simulink model "dng_aircraft_demo"  (Simulink 5.0)
settings: Solver=ode45  StartTime=0.0  StopTime=inf  MaxStep=0.1  RelTol=1e-2  AbsTol=1e-3
PreLoadFcn:
  | load dng_aircraft_init;
values from neighbouring files (symbols this model uses):
  AM = [-0.03554 -0.002226 -0.05504 0.000591 0.09448 -0.003117 0.00292 0 -5.578 0 -0.6028 0 ... (114 elements, 6x19)]    [dng_aircraft_init.mat]
  GM1 = [1.5875 14.63 23.23 5368.39 6928.93 11158.75 0 117.64 0 2288.231]    [dng_aircraft_init.mat]
  uaero0 = [-0.0317656979071 -0.0320210159663 -0.0365180369264 0]    [dng_aircraft_init.mat]
  uprop0 = [1800 22.5734756773]    [dng_aircraft_init.mat]
  xfix = 1    [dng_aircraft_init.mat]
  xinco = [45 0.13029612885 0.0603452248515 0 0 0 0 0.13029612885 0 0 0 1000]    [dng_aircraft_init.mat]
undefined symbols (not defined in the file or in its folder): tcinclinometer, tcturn, xpos, ypos, zpos
libraries: dnglibv1 x10
settings Model: Creator=nikita  LastModifiedBy=howie  ExtModeTrigMode=oneshot  ExtModeArmWhenConnect=off  LimitDataPoints=off  IntegerOverflowMsg=none  BlockReductionOpt=off  BooleanDataType=off
settings Model: ModifiedHistory=|
  | March 03, 1999:
  | Fine-tuned control parameters. Included rate-limiter in flap-signal.
  | Included 1st-order lag filter in vertical speed signal. - Marc Rauw.

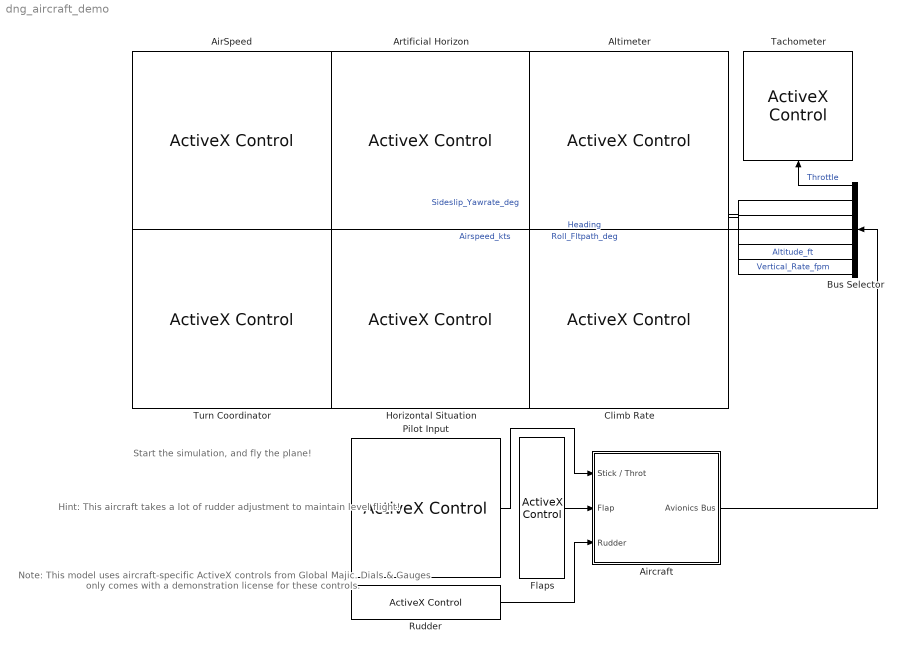
== system dng_aircraft_demo ==
  note: Note: This model uses
      | aircraft-specific ActiveX
      | controls from Global Majic.
      | Dials & Gauges only comes
      | with a demonstration
      | license for these controls.
  note: Start the simulation,
      | and fly the plane!
  note: Hint: This aircraft takes a
      | lot of rudder adjustment
      | to maintain level flight!
  AirSpeed : dnglibv1/ActiveX Control  Orientation=up  progid=air.airctrl.1  connect=input  input=airspeed  init=hActx.displaymode=4;  inblock=on  border=off  dialOut=0  updateParam=0
  Aircraft : Subsystem
  Altimeter : dnglibv1/ActiveX Control  Orientation=up  progid=air.airctrl.1  connect=input  input=altitude  init=hActx.displaymode=2;hActx.altthousandstyle=1;  inblock=on  border=off  dialOut=0  updateParam=0
  Artificial Horizon : dnglibv1/ActiveX Control  Orientation=up  progid=air.airctrl.1  connect=input  input=ahroll, ahpitch  init=hActx.displaymode=6;  inblock=on  border=off  dialOut=0  updateParam=0
  Bus Selector : BusSelector  Orientation=left  OutputSignals=Throttle,Avionics.Airspeed_kts,Avionics.Roll_Fltpath_deg,Avionics.Sideslip_Yawrate_deg,Avionics.Heading,Avionics.Altitude_ft,Avionics.Vertical_Rate_fpm
  Climb Rate : dnglibv1/ActiveX Control  Orientation=down  progid=air.airctrl.1  connect=input  input=climbrate  init=hActx.displaymode=3;  inblock=on  border=off  dialOut=0  updateParam=0
  Flaps : dnglibv1/ActiveX Control  progid=mwslider.sliderctrl.1  connect=output  output=value  dialOutEvent=Slide  init=hActx.configuration='Slider\Basic\Vertical\Simple Slider 3';dng_aircraft_set_flap(hActx);  inblock=on  border=off  dialOut=1  updateParam=0
  Horizontal Situation : dnglibv1/ActiveX Control  Orientation=down  progid=air.airctrl.1  connect=input  input=hsiheading  init=hActx.displaymode=5;  inblock=on  border=off  dialOut=0  updateParam=0
  Pilot Input : dnglibv1/ActiveX Control  progid=JOYSTICK.JoystickCtrl.1  connect=output  output=ypos,xpos,zpos  dialOutEvent=JoyMove  init=hActx.displaymode=1;hActx.ymax=-9; hActx.ymin=9; hActx.xmax=-18;hActx.xmin=18;hActx.zmin=2600; hActx.zmax=1100;hActx.zpos=1800;  inblock=on  border=off  dialOut=[0.000176597852259874;1.4586243135349e-019;1800]  updateParam=0
  Rudder : dnglibv1/ActiveX Control  progid=mwslider.sliderctrl.1  connect=output  output=value  dialOutEvent=Slide  init=hActx.configuration='Slider\Basic\Horizontal\Simple Slider3';hActx.min=-5;hActx.max=5;hActx.value=0;  inblock=on  border=off  dialOut=0  updateParam=0
  Tachometer : dnglibv1/ActiveX Control  Orientation=up  progid=mwagauge.agaugectrl.1  connect=input  input=NeedleValue  init=hActx.configuration='Angular Gauge\Automobile Instruments\Engine RPM';hActx.scalemaxvalue=5000;hActx.Tics=1;hActx.TicAutoTic=1;hActx.TicAutoCount=4;hActx.Captions=1;hActx.Caption='RPM';  inblock=on  border=off  dialOut=0  updateParam=0
  Turn Coordinator : dnglibv1/ActiveX Control  Orientation=down  progid=air.airctrl.1  connect=input  input=tcinclinometer,tcturn  init=hActx.displaymode=7;  inblock=on  border=off  dialOut=0  updateParam=0
  wires:
  Aircraft/1(Avionics Bus) -> Bus Selector/1
  Bus Selector/2 -> AirSpeed/1  "Airspeed_kts"
  Bus Selector/3 -> Artificial Horizon/1  "Roll_Fltpath_deg"
  Bus Selector/5 -> Horizontal Situation/1  "Heading"
  Bus Selector/6 -> Altimeter/1  "Altitude_ft"
  Bus Selector/7 -> Climb Rate/1  "Vertical_Rate_fpm"
  Pilot Input/1 -> Aircraft/1(Stick / Throt)
  Rudder/1 -> Aircraft/3(Rudder)
  Flaps/1 -> Aircraft/2(Flap)
  Bus Selector/4 -> Turn Coordinator/1  "Sideslip_Yawrate_deg"
  Bus Selector/1 -> Tachometer/1  "Throttle"

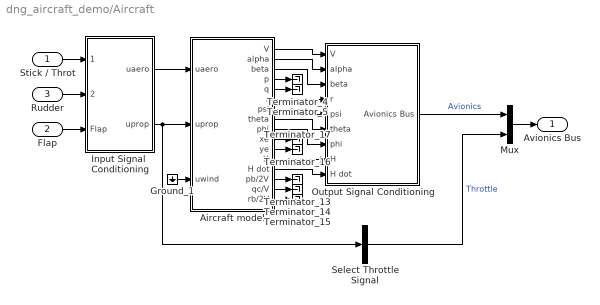
== system dng_aircraft_demo/Aircraft ==
  Stick / Throt : Inport
  Flap : Inport  Port=2
  Rudder : Inport  Port=3
  Aircraft model : Subsystem
  Ground_1 : Ground
  Input Signal  Conditioning : Subsystem
  Mux : Mux  Inputs=2
  Output Signal Conditioning : Subsystem
  Select Throttle Signal : BusSelector  OutputSignals=Throttle
  Terminator_{4..5,13..17} (7 alike) : Terminator
  Avionics Bus : Outport
  wires:
  Input Signal  Conditioning/1(uaero) -> Aircraft model/1(uaero)
  Ground_1/1 -> Aircraft model/3(uwind)
  Stick / Throt/1 -> Input Signal  Conditioning/1(Stick / Throt)
  Rudder/1 -> Input Signal  Conditioning/2(Rudder)
  Flap/1 -> Input Signal  Conditioning/3(Flap)
  Aircraft model/4(p) -> Terminator_4/1
  Aircraft model/5(q) -> Terminator_5/1
  Aircraft model/10(xe) -> Terminator_16/1
  Aircraft model/11(ye) -> Terminator_17/1
  Aircraft model/14(pb/2V) -> Terminator_13/1
  Aircraft model/15(qc/V) -> Terminator_14/1
  Aircraft model/16(rb/2V) -> Terminator_15/1
  Aircraft model/1(V) -> Output Signal Conditioning/1(V)
  Aircraft model/2(alpha) -> Output Signal Conditioning/2(alpha)
  Aircraft model/3(beta) -> Output Signal Conditioning/3(beta)
  Aircraft model/6(r) -> Output Signal Conditioning/4(r)
  Aircraft model/7(psi) -> Output Signal Conditioning/5(psi)
  Aircraft model/8(theta) -> Output Signal Conditioning/6(theta)
  Aircraft model/9(phi) -> Output Signal Conditioning/7(phi)
  Aircraft model/12(H) -> Output Signal Conditioning/8(H)
  Aircraft model/13(H dot) -> Output Signal Conditioning/9(H dot)
  Mux/1 -> Avionics Bus/1
  Output Signal Conditioning/1(Avionics Bus) -> Mux/1  "Avionics"
  Input Signal  Conditioning/2(uprop) -> Aircraft model/2(uprop), Select Throttle Signal/1
  Select Throttle Signal/1 -> Mux/2  "Throttle"

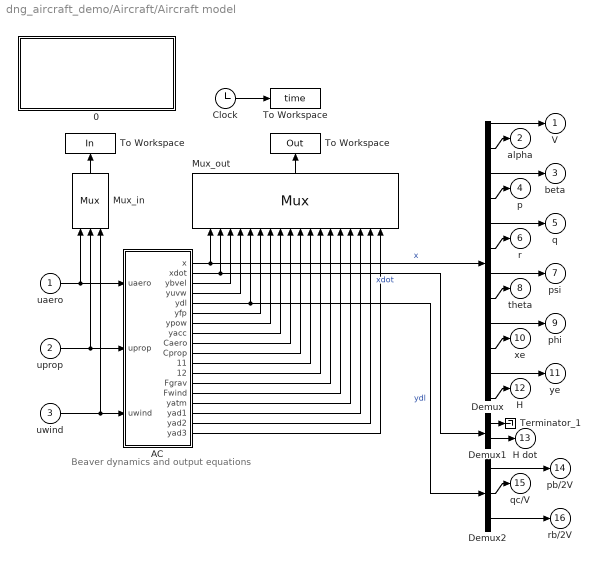
== system dng_aircraft_demo/Aircraft/Aircraft model ==
  note: Beaver dynamics
      | and output equations
  uaero : Inport  PortDimensions=4
  uprop : Inport  Port=2  PortDimensions=2
  uwind : Inport  Port=3  PortDimensions=6
  0 : Subsystem
      settings: OpenFcn=web('http://callisto.worldonline.nl/~rauw');
      mask Display: disp('Dynamic model of the\nDe Havilland DHC-2 ''Beaver'',\ncreated by M.O. Rauw.\nDouble-click for more info.')
  AC : Subsystem
  Clock : Clock
      settings: Decimation=10
  Demux : Demux  Outputs=12
  Demux1 : Demux  Outputs=[11 1]
  Demux2 : Demux  Outputs=3
  Mux_in : Mux  Orientation=up  Inputs=[4 2 6]
      settings: OpenFcn=web('http://callisto.worldonline.nl/~rauw');
      mask Display: disp('Mux\nClick\n2x for\ninfo!')
  Mux_out : Mux  Orientation=up  Inputs=[12 12 3 3 3 4 2 6 6 6 6 6 3 3 5 3 3 3]
      settings: OpenFcn=web('http://callisto.worldonline.nl/~rauw');
      mask Display: disp('Mux\n\nDouble-click for more info!')
  Terminator_1 : Terminator
  To Workspace : ToWorkspace  VariableName=Out  SaveFormat=Array
      settings: Orientation=up  MaxDataPoints=5000
  "To Workspace " : ToWorkspace  VariableName=In  SaveFormat=Array
      settings: Orientation=up  MaxDataPoints=5000
  "To Workspace  " : ToWorkspace  VariableName=time  SaveFormat=Array
      settings: MaxDataPoints=5000
  V : Outport  InitialOutput=0
  alpha : Outport  Port=2  InitialOutput=0
  beta : Outport  Port=3  InitialOutput=0
  p : Outport  Port=4  InitialOutput=0
  q : Outport  Port=5  InitialOutput=0
  r : Outport  Port=6  InitialOutput=0
  psi : Outport  Port=7  InitialOutput=0
  theta : Outport  Port=8  InitialOutput=0
  phi : Outport  Port=9  InitialOutput=0
  xe : Outport  Port=10  InitialOutput=0
  ye : Outport  Port=11  InitialOutput=0
  H : Outport  Port=12  InitialOutput=0
  H dot : Outport  Port=13  InitialOutput=0
  pb/2V : Outport  Port=14  InitialOutput=0
  qc/V : Outport  Port=15  InitialOutput=0
  rb/2V : Outport  Port=16  InitialOutput=0
  wires:
  uaero/1 -> Mux_in/1, AC/1(uaero)
  uprop/1 -> Mux_in/2, AC/2(uprop)
  uwind/1 -> Mux_in/3, AC/3(" uwind")
  AC/18(yad3) -> Mux_out/18
  AC/17(yad2) -> Mux_out/17
  AC/4(yuvw) -> Mux_out/4
  AC/1(x) -> Mux_out/1, Demux/1  "x"
  AC/3(ybvel) -> Mux_out/3
  AC/16(yad1) -> Mux_out/16
  AC/5(ydl) -> Mux_out/5, Demux2/1  "ydl"
  AC/6(yfp) -> Mux_out/6
  AC/8(yacc) -> Mux_out/8
  AC/9(Caero) -> Mux_out/9
  AC/10(Cprop) -> Mux_out/10
  AC/11(FMaero) -> Mux_out/11
  AC/12(FMprop) -> Mux_out/12
  AC/13(Fgrav) -> Mux_out/13
  AC/14(Fwind) -> Mux_out/14
  AC/15(yatm) -> Mux_out/15
  AC/2(xdot) -> Demux1/1, Mux_out/2  "xdot"
  Demux2/3 -> rb/2V/1
  Demux2/2 -> qc/V/1
  Demux2/1 -> pb/2V/1
  Demux1/2 -> H dot/1
  Demux/10 -> xe/1
  Demux/11 -> ye/1
  Demux/12 -> H/1
  Demux/9 -> phi/1
  Demux/8 -> theta/1
  Demux/7 -> psi/1
  Demux/6 -> r/1
  Demux/5 -> q/1
  Demux/4 -> p/1
  Demux/3 -> beta/1
  Demux/2 -> alpha/1
  Demux/1 -> V/1
  Demux1/1 -> Terminator_1/1
  Clock/1 -> "To Workspace  "/1
  Mux_out/1 -> To Workspace/1
  Mux_in/1 -> "To Workspace "/1
  AC/7(ypow) -> Mux_out/7

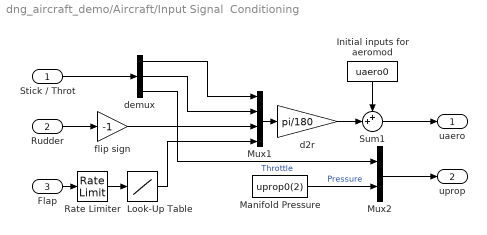
== system dng_aircraft_demo/Aircraft/Input Signal  Conditioning ==
  Stick / Throt : Inport
  Rudder : Inport  Port=2
  Flap : Inport  Port=3
  Initial inputs for aeromod : Constant  Orientation=down  Value=uaero0
  Look-Up Table : Lookup  InputValues=[0:3]  OutputValues=[0 4 10 20]  SaturateOnIntegerOverflow=on
  Manifold Pressure : Constant  Value=uprop0(2)
  Mux1 : Mux
  Mux2 : Mux  Inputs=2
  Rate Limiter : RateLimiter  RisingSlewLimit=0.5  FallingSlewLimit=-0.5
  Sum1 : Sum  Inputs=++|  SaturateOnIntegerOverflow=on  InputSameDT=on
  d2r : Gain  Gain=pi/180  SaturateOnIntegerOverflow=on
  demux : Demux  Outputs=3
  flip sign : Gain  Gain=-1  SaturateOnIntegerOverflow=on
  uaero : Outport
  uprop : Outport  Port=2
  wires:
  Sum1/1 -> uaero/1
  Mux2/1 -> uprop/1
  Initial inputs for aeromod/1 -> Sum1/1
  Mux1/1 -> d2r/1
  d2r/1 -> Sum1/2
  flip sign/1 -> Mux1/3
  Manifold Pressure/1 -> Mux2/2  "Pressure"
  demux/2 -> Mux1/2
  demux/1 -> Mux1/1
  demux/3 -> Mux2/1  "Throttle"
  Look-Up Table/1 -> Mux1/4
  Rudder/1 -> flip sign/1
  Stick / Throt/1 -> demux/1
  Rate Limiter/1 -> Look-Up Table/1
  Flap/1 -> Rate Limiter/1

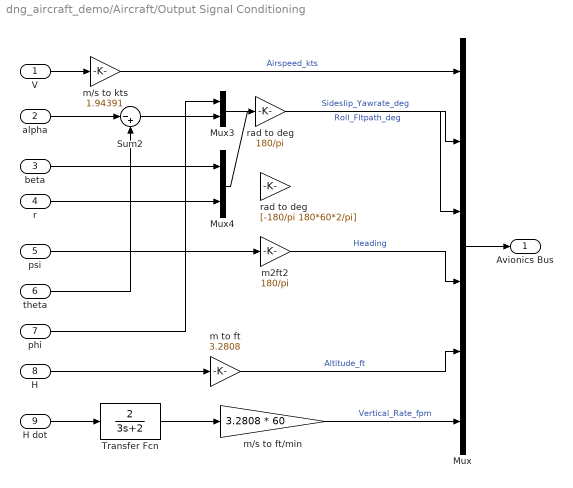
== system dng_aircraft_demo/Aircraft/Output Signal Conditioning ==
  V : Inport
  alpha : Inport  Port=2
  beta : Inport  Port=3
  r : Inport  Port=4
  psi : Inport  Port=5
  theta : Inport  Port=6
  phi : Inport  Port=7
  H : Inport  Port=8
  H dot : Inport  Port=9
  Mux : Mux  Inputs=6
  Mux3 : Mux  Inputs=2
  Mux4 : Mux  Inputs=2
  Sum2 : Sum  Inputs=|-+  SaturateOnIntegerOverflow=on  InputSameDT=on
  Transfer Fcn : TransferFcn  Numerator=[2]  Denominator=[3 2]
  m to ft : Gain  Gain=3.2808  SaturateOnIntegerOverflow=on
  m/s to kts : Gain  Gain=1.94391  SaturateOnIntegerOverflow=on
  m/s to ft/min : Gain  Gain=3.2808 * 60  SaturateOnIntegerOverflow=on
  m2ft2 : Gain  Gain=180/pi  SaturateOnIntegerOverflow=on
  rad to deg : Gain  Gain=180/pi  SaturateOnIntegerOverflow=on
  rad to deg : Gain  Gain=[-180/pi 180*60*2/pi]  SaturateOnIntegerOverflow=on
  Avionics Bus : Outport
  wires:
  H/1 -> m to ft/1
  V/1 -> m/s to kts/1
  alpha/1 -> Sum2/1
  theta/1 -> Sum2/2
  beta/1 -> Mux4/1
  r/1 -> Mux4/2
  Mux4/1 -> rad to deg/1
  phi/1 -> Mux3/1
  Sum2/1 -> Mux3/2
  Mux3/1 -> rad to deg/1
  psi/1 -> m2ft2/1
  Mux/1 -> Avionics Bus/1
  m to ft/1 -> Mux/5  "Altitude_ft"
  m2ft2/1 -> Mux/4  "Heading"
  rad to deg/1 -> Mux/3  "Sideslip_Yawrate_deg"
  rad to deg/1 -> Mux/2  "Roll_Fltpath_deg"
  m/s to kts/1 -> Mux/1  "Airspeed_kts"
  m/s to ft/min/1 -> Mux/6  "Vertical_Rate_fpm"
  H dot/1 -> Transfer Fcn/1
  Transfer Fcn/1 -> m/s to ft/min/1

== system dng_aircraft_demo/Aircraft/Aircraft model/0 ==

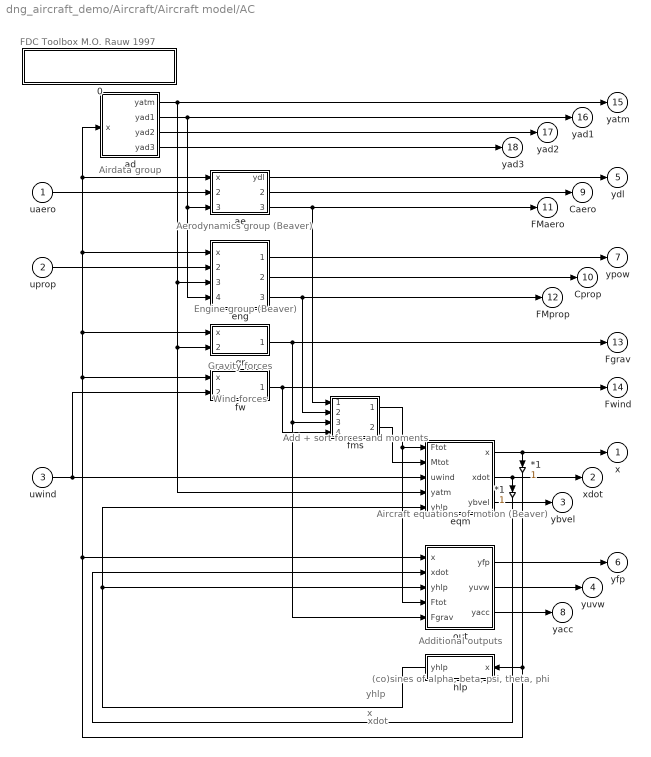
== system dng_aircraft_demo/Aircraft/Aircraft model/AC ==
  note: Airdata group
  note: Add + sort
      | forces and
      | moments
  note: (co)sines of
      | alpha, beta,
      | psi, theta, phi
  note: Aerodynamics
      | group (Beaver)
  note: Engine group (Beaver)
  note: Gravity forces
  note: Wind forces
  note: Aircraft equations
      | of motion (Beaver)
  note: Additional outputs
  note: yhlp
  note: x
  note: xdot
  note: FDC Toolbox
      |  M.O. Rauw 1997
  uaero : Inport
  uprop : Inport  Port=2
  " uwind" : Inport  Port=3
  " *1" : Gain  Orientation=down  SaturateOnIntegerOverflow=on
  *1 : Gain  Orientation=down  SaturateOnIntegerOverflow=on
  0 : Subsystem
      settings: OpenFcn=web('http://callisto.worldonline.nl/~rauw');
      mask Display: disp('BEAVER, level 2 (main level)\nM.O. Rauw')
  ad : Subsystem
  ae : Subsystem
  eng : Subsystem
  eqm : Subsystem
  fms : Subsystem
      mask Type: FMsort
      mask Description: Forces and Moments sorting block
      mask Help: web('http://callisto.worldonline.nl/~rauw');
      mask Display: disp('FMsort')
  fw : Subsystem  mask(fwind){m=GM1(10)}
      mask prompts: m "Mass of the aircraft [kg]:"
      mask help: Forces due to non-steady atmosphere.
      mask Help: web('http://callisto.worldonline.nl/~rauw');
      mask Display: disp('Fwind')
  gr : Subsystem  mask(Gravity){m=GM1(10)}
      mask prompts: m "Mass of the aircraft [kg]:"
      mask help: Gravity forces.
      mask Help: web('http://callisto.worldonline.nl/~rauw');
      mask Display: disp('Gravity')
  hlp : Subsystem  Orientation=left
      mask Type: Hlpfcn
      mask Description: Help sines and cosines
      mask Help: web('http://callisto.worldonline.nl/~rauw');
      mask Display: disp('hlpfcn')
  out : Subsystem
  x : Outport  InitialOutput=0
  xdot : Outport  Port=2  InitialOutput=0
  ybvel : Outport  Port=3  InitialOutput=0
  yuvw : Outport  Port=4  InitialOutput=0
  ydl : Outport  Port=5  InitialOutput=0
  yfp : Outport  Port=6  InitialOutput=0
  ypow : Outport  Port=7  InitialOutput=0
  yacc : Outport  Port=8  InitialOutput=0
  Caero : Outport  Port=9  InitialOutput=0
  Cprop : Outport  Port=10  InitialOutput=0
  FMaero : Outport  Port=11  InitialOutput=0
  FMprop : Outport  Port=12  InitialOutput=0
  Fgrav : Outport  Port=13  InitialOutput=0
  Fwind : Outport  Port=14  InitialOutput=0
  yatm : Outport  Port=15  InitialOutput=0
  yad1 : Outport  Port=16  InitialOutput=0
  yad2 : Outport  Port=17  InitialOutput=0
  yad3 : Outport  Port=18  InitialOutput=0
  wires:
  fms/2(Mtot) -> eqm/2(Mtot)
  fms/1(Ftot) -> eqm/1(Ftot), out/4(Ftot)
  eqm/1(x) -> " *1"/1, x/1
  eqm/2(xdot) -> *1/1, xdot/1
  " *1"/1 -> ad/1(x), ae/1(x), eng/1(x), gr/1(x), fw/1(x), out/1(x), hlp/1(x)
  gr/1(Fgrav) -> out/5(Fgrav), fms/3(Fgrav), Fgrav/1
  *1/1 -> out/2(xdot)
  " uwind"/1 -> fw/2(uwind), eqm/3(uwind)
  hlp/1(yhlp) -> out/3(yhlp), eqm/5(yhlp)
  ae/3(FMaero) -> fms/1(FMaero), FMaero/1
  eng/3(FMprop) -> fms/2(FMprop), FMprop/1
  fw/1(Fwind) -> fms/4(Fwind), Fwind/1
  out/3(yacc) -> yacc/1
  ad/1(yatm) -> gr/2(yatm), eqm/4(yatm), eng/3(yatm), yatm/1
  ad/3(yad2) -> yad2/1
  ad/2(yad1) -> yad1/1, ae/3(yad1), eng/4(yad1)
  out/1(yfp) -> yfp/1
  eqm/3(ybvel) -> ybvel/1
  eng/2(Cprop) -> Cprop/1
  eng/1(ypow) -> ypow/1
  ae/2(Caero) -> Caero/1
  ae/1(ydl) -> ydl/1
  ad/4(yad3) -> yad3/1
  uaero/1 -> ae/2(uaero)
  uprop/1 -> eng/2(uprop)
  out/2(yuvw) -> yuvw/1

== system dng_aircraft_demo/Aircraft/Aircraft model/AC/0 ==

== system dng_aircraft_demo/Aircraft/Aircraft model/AC/ad ==
  x : Inport
  0 : Subsystem
      settings: OpenFcn=web('http://callisto.worldonline.nl/~rauw');
      mask Display: disp('AIRDATA GROUP (level 3)\nM.O. Rauw')
  ad1 : Subsystem
      mask Type: Airdata1
      mask Description: Basic airdata variables
      mask Help: web('http://callisto.worldonline.nl/~rauw');
      mask Display: disp('Airdata1')
  ad2 : Subsystem
      mask Type: Airdata2
      mask Description: More airdata variables
      mask Help: web('http://callisto.worldonline.nl/~rauw');
      mask Display: disp('Airdata2')
  ad3 : Subsystem  mask(Airdata3){cbar=GM1(1)}
      mask prompts: cbar "Mean aerodynamic chord [m]:"
      mask help: More airdata variables
      mask Help: web('http://callisto.worldonline.nl/~rauw');
      mask Display: disp('Airdata3')
  atm : Subsystem
      mask Type: Atmosph
      mask Description: Atmosphere variables
      mask Help: web('http://callisto.worldonline.nl/~rauw');
      mask Display: disp('Atmosph')
  yatm : Outport  InitialOutput=0
  yad1 : Outport  Port=2  InitialOutput=0
  yad2 : Outport  Port=3  InitialOutput=0
  yad3 : Outport  Port=4  InitialOutput=0
  wires:
  ad1/1(yad1) -> ad3/3(yad1), ad2/2(yad1), yad1/1
  atm/1(yatm) -> ad3/2(yatm), ad2/1(yatm), ad1/2(yatm), yatm/1
  x/1 -> ad3/1(x), ad1/1(x), atm/1(x)
  ad3/1(yad3) -> yad3/1
  ad2/1(yad2) -> yad2/1

== system dng_aircraft_demo/Aircraft/Aircraft model/AC/ae ==
  x : Inport
  uaero : Inport  Port=2
  yad1 : Inport  Port=3
  0 : Subsystem
      settings: OpenFcn=web('http://callisto.worldonline.nl/~rauw');
      mask Display: disp('AERODYNAMICS GROUP (level 3)\nM.O. Rauw')
  aero : Subsystem
      mask Type: Aeromod
      mask Description: Aerodynamic model of the DHC-2 'Beaver'.
      mask Help: web('http://callisto.worldonline.nl/~rauw');
      mask Display: disp('Aeromod\n(Beaver)')
  dl : Subsystem  mask(Dimless){cbar=GM1(1), b=GM1(2)}
      mask prompts: cbar "Mean aerodynamic chord [m]:"; b "Wing span [m]:"
      mask help: Dimensionless rotational velocities.
      mask Help: web('http://callisto.worldonline.nl/~rauw');
      mask Display: disp('Dimless')
  fmdims : Subsystem  mask(FMdims){cbar=GM1(1), b=GM1(2), S=GM1(3)}
      mask prompts: cbar "Mean aerodynamic chord [m]:"; b "Wing span [m]:"; S "Wing surface [m^2]:"
      mask help:
      | Calculate forces and moments from
      | dimensionless coefficients.
      mask Help: web('http://callisto.worldonline.nl/~rauw');
      mask Display: disp('FMdims')
  ydl : Outport  InitialOutput=0
  Caero : Outport  Port=2  InitialOutput=0
  FMaero : Outport  Port=3  InitialOutput=0
  wires:
  fmdims/1(Forces and moments) -> FMaero/1
  yad1/1 -> fmdims/1(yad1)
  uaero/1 -> aero/2(uaero)
  x/1 -> aero/1(x), dl/1(x)
  dl/1(ydl) -> aero/3(ydl), ydl/1
  aero/1(Caero) -> fmdims/2(Force / moment coefficients), Caero/1

== system dng_aircraft_demo/Aircraft/Aircraft model/AC/eng ==
  x : Inport
  uprop : Inport  Port=2
  yatm : Inport  Port=3
  yad1 : Inport  Port=4
  0 : Subsystem
      settings: OpenFcn=web('http://callisto.worldonline.nl/~rauw');
      mask Display: disp('ENGINE GROUP (level 3)\nM.O. Rauw')
  eng : Subsystem
      mask Type: Engmod
      mask Description: Engine model for the DHC-2 'Beaver'
      mask Help: web('http://callisto.worldonline.nl/~rauw');
      mask Display: disp('Engmod\n(Beaver)')
  fmdims : Subsystem  mask(FMdims){cbar=GM1(1), b=GM1(2), S=GM1(3)}
      mask prompts: cbar "Mean aerodynamic chord [m]:"; b "Wing span [m]:"; S "Wing surface [m^2]:"
      mask help:
      | Calculate forces and moments from
      | dimensionless coefficients.
      mask Help: web('http://callisto.worldonline.nl/~rauw');
      mask Display: disp('FMdims')
  pow : Subsystem
      mask Type: Power
      mask Description:
      | Engine power and dimensionless
      | pressure increase across propeller
      | (model for DHC-2 'Beaver')
      mask Help: web('http://callisto.worldonline.nl/~rauw');
      mask Display: disp('Power\n(Beaver)')
  ypow : Outport  InitialOutput=0
  Cprop : Outport  Port=2  InitialOutput=0
  FMprop : Outport  Port=3  InitialOutput=0
  wires:
  yatm/1 -> pow/3(yatm)
  x/1 -> eng/1(x), pow/1(x)
  yad1/1 -> fmdims/1(yad1)
  eng/1(Cprop) -> fmdims/2(Force / moment coefficients), Cprop/1
  fmdims/1(Forces and moments) -> FMprop/1
  uprop/1 -> pow/2(uprop)
  pow/1(ypow) -> eng/2(ypow), ypow/1

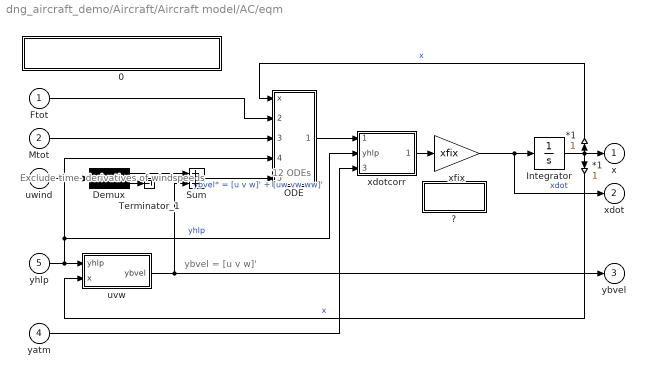
== system dng_aircraft_demo/Aircraft/Aircraft model/AC/eqm ==
  note: ybvel = [u v w]'
  note: Exclude time-
      | derivatives
      | of windspeeds
  note: 12 ODEs
  Ftot : Inport
  Mtot : Inport  Port=2
  uwind : Inport  Port=3
  yatm : Inport  Port=4
  yhlp : Inport  Port=5
  " *1" : Gain  Orientation=up  SaturateOnIntegerOverflow=on
  *1 : Gain  Orientation=down  SaturateOnIntegerOverflow=on
  0 : Subsystem
      settings: OpenFcn=web('http://callisto.worldonline.nl/~rauw');
      mask Display: disp('EQUATIONS OF MOTION (level 3)\nM.O. Rauw')
  "?" : Subsystem
      settings: OpenFcn=web('http://callisto.worldonline.nl/~rauw');
      mask Display: disp('More info\nfor xfix')
  Demux : Demux  Outputs=[3 3]
  Integrator : Integrator  InitialCondition=xinco
  ODE : Subsystem
  Sum : Sum  SaturateOnIntegerOverflow=on  InputSameDT=on
  Terminator_1 : Terminator
  uvw : Subsystem
      mask Type: uvw
      mask Description:
      | Calculation of body-axes velocities
      | u, v, and w
      mask Help: web('http://callisto.worldonline.nl/~rauw');
      mask Display: disp('Body-axes\nvelocities')
  xdotcorr : Subsystem  mask(xdotcorr){b=GM1(2), S=GM1(3), m=GM1(10), CYbdot=AM(2,19)}
      mask prompts: b "Wing span [m]:"; S "Wing surface [m^2]:"; m "Mass of the aircraft [kg]:"; CYbdot "Stability-derivative CYbdot:"
      mask help:
      | Correction block to write state
      | equations for DHC-2 Beaver aircraft
      | explicitly.
      mask Help: web('http://callisto.worldonline.nl/~rauw');
      mask Display: disp('xdotcorr\n(Beaver)')
  xfix : Gain  Gain=xfix  SaturateOnIntegerOverflow=on
  x : Outport  InitialOutput=0
  xdot : Outport  Port=2  InitialOutput=0
  ybvel : Outport  Port=3  InitialOutput=0
  wires:
  Demux/2 -> Terminator_1/1
  yhlp/1 -> uvw/1(yhlp), ODE/4(yhlp), xdotcorr/2(yhlp)  "yhlp"
  ODE/1(xdot) -> xdotcorr/1(xdot uncorrected)
  Sum/1 -> ODE/5(ybvel*)  "ybvel* = [u v w]' + [uw vw ww]'"
  uvw/1(ybvel) -> ybvel/1, Sum/2
  uwind/1 -> Demux/1
  Demux/1 -> Sum/1
  xdotcorr/1(xdot corrected) -> xfix/1
  yatm/1 -> xdotcorr/3(yatm)
  Ftot/1 -> ODE/2(Ftot)
  Mtot/1 -> ODE/3(Mtot)
  *1/1 -> uvw/2(x)  "x"
  Integrator/1 -> x/1, " *1"/1, *1/1
  xfix/1 -> Integrator/1, xdot/1  "xdot"
  " *1"/1 -> ODE/1(x)  "x"

== system dng_aircraft_demo/Aircraft/Aircraft model/AC/fms ==
  note: `
  FMaero : Inport
  FMprop : Inport  Port=2
  Fgrav : Inport  Port=3
  Fwind : Inport  Port=4
  0 : Subsystem
      settings: OpenFcn=web('http://callisto.worldonline.nl/~rauw');
      mask Display: disp('FMSORT\nM.O. Rauw, October 1997')
  Demux : Demux  Outputs=[3 3]
  Demux1 : Demux  Outputs=[3 3]
  Sum1 : Sum  SaturateOnIntegerOverflow=on  InputSameDT=on
  Sum3 : Sum  Inputs=++++  SaturateOnIntegerOverflow=on  InputSameDT=on
  Ftot : Outport  InitialOutput=0
  Mtot : Outport  Port=2  InitialOutput=0
  wires:
  Fwind/1 -> Sum3/4
  Demux/1 -> Sum3/1
  Sum1/1 -> Mtot/1
  Sum3/1 -> Ftot/1
  Demux1/1 -> Sum3/2
  Fgrav/1 -> Sum3/3
  Demux/2 -> Sum1/1
  Demux1/2 -> Sum1/2
  FMprop/1 -> Demux1/1
  FMaero/1 -> Demux/1

== system dng_aircraft_demo/Aircraft/Aircraft model/AC/fw ==
  x : Inport
  uwind : Inport  Port=2
  -Xw/m : Fcn  Expr=u[16] + u[5]*u[15] - u[6]*u[14]
  -Yw/m : Fcn  Expr=u[17] - u[4]*u[15] + u[6]*u[13]
  -Zw/m : Fcn  Expr=u[18] + u[4]*u[14] - u[5]*u[13]
  0 : Subsystem
      settings: OpenFcn=web('http://callisto.worldonline.nl/~rauw');
      mask Display: disp('FWIND\nM.O. Rauw, Dec. 1996')
  Mux : Mux  Inputs=3
  Mux1 : Mux  Inputs=[12 6]
  gain : Gain  Gain=-m  SaturateOnIntegerOverflow=on
  Fwind : Outport  InitialOutput=0
  wires:
  -Zw/m/1 -> Mux/3
  -Xw/m/1 -> Mux/1
  -Yw/m/1 -> Mux/2
  Mux1/1 -> -Xw/m/1, -Zw/m/1, -Yw/m/1
  Mux/1 -> gain/1
  gain/1 -> Fwind/1
  x/1 -> Mux1/1
  uwind/1 -> Mux1/2

== system dng_aircraft_demo/Aircraft/Aircraft model/AC/gr ==
  x : Inport
  yatm : Inport  Port=2
  0 : Subsystem
      settings: OpenFcn=web('http://callisto.worldonline.nl/~rauw');
      mask Display: disp('GRAVITY\nM.O. Rauw, October 1997')
  Mux : Mux  Inputs=3
  Mux1 : Mux  Inputs=[12 5]
  Xgr : Fcn  Expr=-m*u[17]*sin(u[8])
  Ygr : Fcn  Expr=m*u[17]*cos(u[8])*sin(u[9])
  Zgr : Fcn  Expr=m*u[17]*cos(u[8])*cos(u[9])
  Fgrav : Outport  InitialOutput=0
  wires:
  yatm/1 -> Mux1/2
  x/1 -> Mux1/1
  Zgr/1 -> Mux/3
  Mux1/1 -> Zgr/1, Xgr/1, Ygr/1
  Mux/1 -> Fgrav/1
  Ygr/1 -> Mux/2
  Xgr/1 -> Mux/1

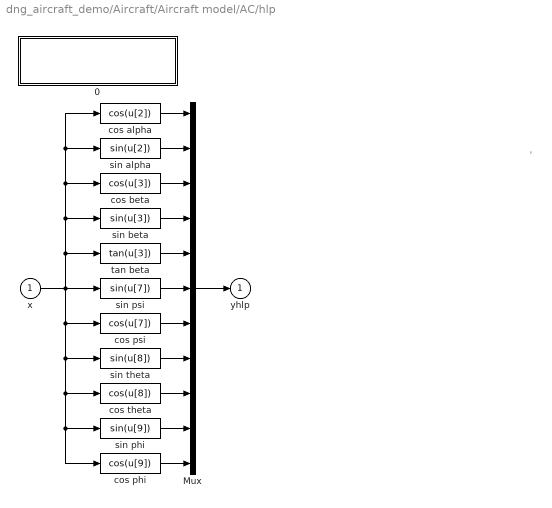
== system dng_aircraft_demo/Aircraft/Aircraft model/AC/hlp ==
  note: '
  x : Inport
  0 : Subsystem
      settings: OpenFcn=web('http://callisto.worldonline.nl/~rauw');
      mask Display: disp('HELP FUNCTIONS\n(often used sines and cosines)\nM.O. Rauw, October 1997')
  Mux : Mux  Inputs=11
  cos alpha : Fcn  Expr=cos(u[2])
  cos beta : Fcn  Expr=cos(u[3])
  cos phi : Fcn  Expr=cos(u[9])
  cos psi : Fcn  Expr=cos(u[7])
  cos theta : Fcn  Expr=cos(u[8])
  sin alpha : Fcn  Expr=sin(u[2])
  sin beta : Fcn  Expr=sin(u[3])
  sin phi : Fcn  Expr=sin(u[9])
  sin psi : Fcn  Expr=sin(u[7])
  sin theta : Fcn  Expr=sin(u[8])
  tan beta : Fcn  Expr=tan(u[3])
  yhlp : Outport  InitialOutput=0
  wires:
  cos phi/1 -> Mux/11
  Mux/1 -> yhlp/1
  sin phi/1 -> Mux/10
  cos theta/1 -> Mux/9
  sin theta/1 -> Mux/8
  cos psi/1 -> Mux/7
  sin psi/1 -> Mux/6
  tan beta/1 -> Mux/5
  sin beta/1 -> Mux/4
  cos beta/1 -> Mux/3
  sin alpha/1 -> Mux/2
  cos alpha/1 -> Mux/1
  x/1 -> cos psi/1, cos phi/1, sin phi/1, cos theta/1, sin theta/1, tan beta/1, cos alpha/1, sin alpha/1, cos beta/1, sin beta/1, sin psi/1

== system dng_aircraft_demo/Aircraft/Aircraft model/AC/out ==
  note: Body-axes accelerations
      | and specific forces
  note: du/dt, dv/dt, dw/dt
      | (output equations!)
  note: Flightpath
      | variables
  x : Inport
  xdot : Inport  Port=2
  yhlp : Inport  Port=3
  Ftot : Inport  Port=4
  Fgrav : Inport  Port=5
  0 : Subsystem
      settings: OpenFcn=web('http://callisto.worldonline.nl/~rauw');
      mask Display: disp('Additional outputs (level 3)\nM.O. Rauw')
  accel : Subsystem  mask(accel){m=GM1(10)}
      mask prompts: m "Mass of the aircraft [kg]:"
      mask help:
      | Body axes accelerations and
      | specific forces.
      mask Help: web('http://callisto.worldonline.nl/~rauw');
      mask Display: disp('Accel')
  fp : Subsystem  mask(Flpath){alpha0=xinco(2)}
      mask prompts: alpha0 "Initial value of angle of attack, alpha0:"
      mask help: Flightpath related parameters.
      mask Help: web('http://callisto.worldonline.nl/~rauw');
      mask Display: disp('flpath')
  uvwdot : Subsystem
      mask Type: uvwdot
      mask Description: Calculation of du/dt, dv/dt, and dw/dt.
      mask Help: web('http://callisto.worldonline.nl/~rauw');
      mask Display: disp('uvwdot')
  yfp : Outport  InitialOutput=0
  yuvw : Outport  Port=2  InitialOutput=0
  yacc : Outport  Port=3  InitialOutput=0
  wires:
  Fgrav/1 -> accel/2(Fgrav)
  x/1 -> uvwdot/1(x), fp/1(x)
  xdot/1 -> uvwdot/2(xdot), fp/2(xdot)
  accel/1(yacc) -> yacc/1
  Ftot/1 -> accel/1(Ftot)
  yhlp/1 -> uvwdot/3(yhlp)
  uvwdot/1(yuvw =  [udot; vdot; wdot]) -> yuvw/1
  fp/1(yfp) -> yfp/1

== system dng_aircraft_demo/Aircraft/Aircraft model/AC/ad/0 ==

== system dng_aircraft_demo/Aircraft/Aircraft model/AC/ad/ad1 ==
  x : Inport
  yatm : Inport  Port=2
  0 : Subsystem
      settings: OpenFcn=web('http://callisto.worldonline.nl/~rauw');
      mask Display: disp('AIRDATA1\nM.O. Rauw, October 1997')
  M : Fcn  Expr=u[2]/u[1]
  Mux : Mux  Inputs=[1 12]
  Mux1 : Mux  Inputs=[12 5]
  Mux2 : Mux  Inputs=3
  a : Fcn  Expr=sqrt(401.8743*u[3])
  qdyn : Fcn  Expr=0.5*u[13]*u[1]^2
  yad1 : Outport  InitialOutput=0
  wires:
  yatm/1 -> Mux1/2, a/1
  x/1 -> Mux1/1, Mux/2
  Mux/1 -> M/1
  Mux1/1 -> qdyn/1
  M/1 -> Mux2/2
  a/1 -> Mux2/1, Mux/1
  qdyn/1 -> Mux2/3
  Mux2/1 -> yad1/1

== system dng_aircraft_demo/Aircraft/Aircraft model/AC/ad/ad2 ==
  yatm : Inport
  yad1 : Inport  Port=2
  0 : Subsystem
      settings: OpenFcn=web('http://callisto.worldonline.nl/~rauw');
      mask Display: disp('AIRDATA2\nM.O. Rauw, October 1997')
  Mux : Mux  Inputs=[5 3]
  Mux1 : Mux  Inputs=3
  Vc : Fcn  Expr=sqrt(579000*((1+u[1]/101325)^(1/3.5)-1))
  Ve : Fcn  Expr=sqrt(u[8] * 1.63265)
  qc : Fcn  Expr=u[2] * ((1+0.2*u[7]^2)^3.5-1)
  yad2 : Outport  InitialOutput=0
  wires:
  Mux1/1 -> yad2/1
  qc/1 -> Mux1/1, Vc/1
  Vc/1 -> Mux1/3
  Ve/1 -> Mux1/2
  Mux/1 -> Ve/1, qc/1
  yatm/1 -> Mux/1
  yad1/1 -> Mux/2

== system dng_aircraft_demo/Aircraft/Aircraft model/AC/ad/ad3 ==
  x : Inport
  yatm : Inport  Port=2
  yad1 : Inport  Port=3
  0 : Subsystem
      settings: OpenFcn=web('http://callisto.worldonline.nl/~rauw');
      mask Display: disp('AIRDATA3\nM.O. Rauw, October 1997')
  Mux : Mux  Inputs=3
  Mux1 : Mux  Inputs=[12 5 3]
  Re : Fcn  Expr=(u[13]*u[1])/u[16]
  Tt : Fcn  Expr=u[15] * (1+0.2*u[19]^2)
  cbar : Gain  Gain=cbar  SaturateOnIntegerOverflow=on
  yad3 : Outport  InitialOutput=0
  wires:
  cbar/1 -> Mux/3
  Tt/1 -> Mux/1
  Mux/1 -> yad3/1
  Mux1/1 -> Tt/1, Re/1
  Re/1 -> cbar/1, Mux/2
  x/1 -> Mux1/1
  yatm/1 -> Mux1/2
  yad1/1 -> Mux1/3

== system dng_aircraft_demo/Aircraft/Aircraft model/AC/ad/atm ==
  x : Inport
  0 : Subsystem
      settings: OpenFcn=web('http://callisto.worldonline.nl/~rauw');
      mask Display: disp('ATMOSPH\nM.O. Rauw, October 1997')
  Mux : Mux  Inputs=2
  Mux1 : Mux  Inputs=[2 1]
  Mux2 : Mux  Inputs=5
  T : Fcn  Expr=288.15 - 0.0065*u[12]
  g : Fcn  Expr=9.80665*(6371020/(6371020+u[12]))^2
  mu : Fcn  Expr=(1.458*10^(-6)*u[2]^1.5)/(u[2]+110.4)
  ps : Fcn  Expr=101325*(u[2]/288.15)^(u[1]/1.86584)
  rho : Fcn  Expr=u[3]/(287.053*u[2])
  yatm : Outport  InitialOutput=0
  wires:
  mu/1 -> Mux2/4
  Mux2/1 -> yatm/1
  Mux1/1 -> rho/1
  rho/1 -> Mux2/1
  g/1 -> Mux2/5, Mux/1
  T/1 -> Mux2/3, Mux/2
  ps/1 -> Mux2/2, Mux1/2
  Mux/1 -> ps/1, mu/1, Mux1/1
  x/1 -> g/1, T/1

== system dng_aircraft_demo/Aircraft/Aircraft model/AC/ae/0 ==

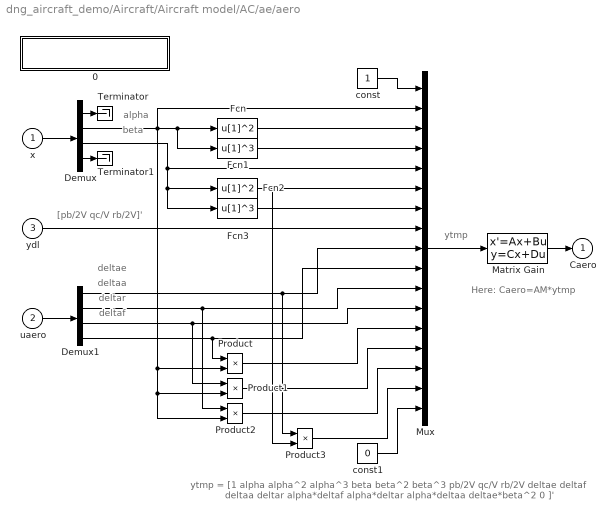
== system dng_aircraft_demo/Aircraft/Aircraft model/AC/ae/aero ==
  note: Here: Caero=AM*ytmp
  note: ytmp
  note: alpha
  note: deltaf
  note: deltar
  note: deltaa
  note: deltae
  note: beta
  note: [pb/2V qc/V rb/2V]'
  note: ytmp = [1  alpha  alpha^2  alpha^3  beta  beta^2  beta^3  pb/2V  qc/V  rb/2V  deltae
      | deltaf  deltaa  deltar  alpha*deltaf  alpha*deltar  alpha*deltaa  deltae*beta^2  0 ]'
  x : Inport
  uaero : Inport  Port=2
  ydl : Inport  Port=3
  0 : Subsystem
      settings: OpenFcn=web('http://callisto.worldonline.nl/~rauw');
      mask Display: disp('AEROMOD\nM.O. Rauw, October 1997')
  Demux : Demux  Outputs=[1 1 1 9]
  Demux1 : Demux
  Fcn : Fcn  Expr=u[1]^2
  Fcn1 : Fcn  Expr=u[1]^3
  Fcn2 : Fcn  Expr=u[1]^2
  Fcn3 : Fcn  Expr=u[1]^3
  Matrix Gain : StateSpace  A=A  B=B  C=C  D=D  mask(Matrix Gain){@1=AM}
      mask prompts: @1 "Gain matrix:"
      mask help: Matrix Gain
      mask init:
      | A = []; B = []; C = []; D = @1;
      mask Help: This block implements an matrix gain.\nThe matrix dimensions must be in accordance\nwith the dimension of the inputvector.
      mask Display: disp('y = A*u')
  Mux : Mux  Inputs=[1 1 1 1 1 1 1 3 1 1 1 1 1 1 1 1 1]
  Product{,1..3} (4 alike) : Product  SaturateOnIntegerOverflow=on  InputSameDT=on
  Terminator : Terminator
  Terminator1 : Terminator
  const : Constant
  const1 : Constant  Value=0
  Caero : Outport  InitialOutput=0
  wires:
  Matrix Gain/1 -> Caero/1
  Mux/1 -> Matrix Gain/1
  x/1 -> Demux/1
  Fcn/1 -> Mux/3
  Fcn1/1 -> Mux/4
  uaero/1 -> Demux1/1
  Fcn3/1 -> Mux/7
  Product/1 -> Mux/13
  Demux1/3 -> Product1/1, Mux/12
  Demux1/2 -> Product2/1, Mux/11
  Demux/3 -> Fcn3/1, Fcn2/1, Mux/5
  Demux/2 -> Product2/2, Product1/2, Product/2, Fcn1/1, Fcn/1, Mux/2
  Demux1/4 -> Product/1, Mux/10
  Fcn2/1 -> Product3/2, Mux/6
  Demux1/1 -> Product3/1, Mux/9
  Product1/1 -> Mux/14
  Product2/1 -> Mux/15
  Product3/1 -> Mux/16
  ydl/1 -> Mux/8
  const/1 -> Mux/1
  const1/1 -> Mux/17
  Demux/1 -> Terminator/1
  Demux/4 -> Terminator1/1

== system dng_aircraft_demo/Aircraft/Aircraft model/AC/ae/dl ==
  x : Inport
  0 : Subsystem
      settings: OpenFcn=web('http://callisto.worldonline.nl/~rauw');
      mask Display: disp('DIMLESS\nM.O. Rauw, October 1997')
  Mux : Mux  Inputs=3
  pb/2V : Fcn  Expr=0.5 * u[4] * b / u[1]
  qc/V : Fcn  Expr=u[5] * cbar / u[1]
  rb/2V : Fcn  Expr=0.5 * u[6] * b / u[1]
  ydl : Outport  InitialOutput=0
  wires:
  x/1 -> pb/2V/1, rb/2V/1, qc/V/1
  Mux/1 -> ydl/1
  rb/2V/1 -> Mux/3
  qc/V/1 -> Mux/2
  pb/2V/1 -> Mux/1

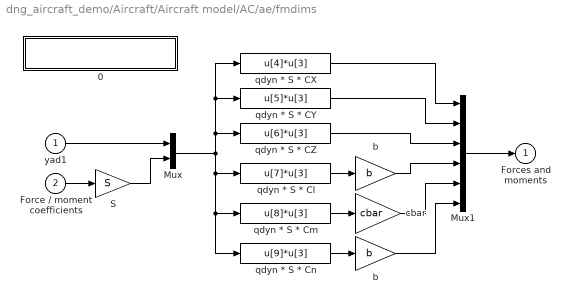
== system dng_aircraft_demo/Aircraft/Aircraft model/AC/ae/fmdims ==
  yad1 : Inport
  Force / moment coefficients : Inport  Port=2
  0 : Subsystem
      settings: OpenFcn=web('http://callisto.worldonline.nl/~rauw');
      mask Display: disp('FMDIMS\nM.O. Rauw, October 1997')
  Mux : Mux  Inputs=[3 6]
  Mux1 : Mux  Inputs=6
  S : Gain  Gain=S  SaturateOnIntegerOverflow=on
  b : Gain  Gain=b  SaturateOnIntegerOverflow=on
  "b " : Gain  Gain=b  SaturateOnIntegerOverflow=on
  cbar : Gain  Gain=cbar  SaturateOnIntegerOverflow=on
  qdyn * S * CX : Fcn  Expr=u[4]*u[3]
  qdyn * S * CY : Fcn  Expr=u[5]*u[3]
  qdyn * S * CZ : Fcn  Expr=u[6]*u[3]
  qdyn * S * Cl : Fcn  Expr=u[7]*u[3]
  qdyn * S * Cm : Fcn  Expr=u[8]*u[3]
  qdyn * S * Cn : Fcn  Expr=u[9]*u[3]
  Forces and moments : Outport  InitialOutput=0
  wires:
  b/1 -> Mux1/4
  qdyn * S * CZ/1 -> Mux1/3
  S/1 -> Mux/2
  qdyn * S * CY/1 -> Mux1/2
  qdyn * S * CX/1 -> Mux1/1
  yad1/1 -> Mux/1
  qdyn * S * Cn/1 -> "b "/1
  qdyn * S * Cm/1 -> cbar/1
  qdyn * S * Cl/1 -> b/1
  Mux/1 -> qdyn * S * Cn/1, qdyn * S * Cm/1, qdyn * S * Cl/1, qdyn * S * CY/1, qdyn * S * CX/1, qdyn * S * CZ/1
  Force / moment coefficients/1 -> S/1
  cbar/1 -> Mux1/5
  "b "/1 -> Mux1/6
  Mux1/1 -> Forces and moments/1

== system dng_aircraft_demo/Aircraft/Aircraft model/AC/eng/0 ==

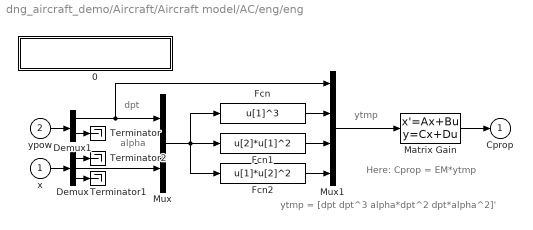
== system dng_aircraft_demo/Aircraft/Aircraft model/AC/eng/eng ==
  note: ytmp
  note: alpha
  note: dpt
  note: ytmp = [dpt dpt^3 alpha*dpt^2 dpt*alpha^2]'
  note: Here: Cprop = EM*ytmp
  x : Inport
  ypow : Inport  Port=2
  0 : Subsystem
      settings: OpenFcn=web('http://callisto.worldonline.nl/~rauw');
      mask Display: disp('ENGMOD\nM.O. Rauw, Dec. 1996')
  Demux : Demux  Outputs=[1 1 10]
  Demux1 : Demux  Outputs=2
  Fcn : Fcn  Expr=u[1]^3
  Fcn1 : Fcn  Expr=u[2]*u[1]^2
  Fcn2 : Fcn  Expr=u[1]*u[2]^2
  Matrix Gain : StateSpace  A=A  B=B  C=C  D=D  mask(Matrix Gain){@1=EM}
      mask prompts: @1 "Gain matrix:"
      mask help: Matrix Gain
      mask init:
      | A = []; B = []; C = []; D = @1;
      mask Help: This block implements an matrix gain.\nThe matrix dimensions must be in accordance\nwith the dimension of the inputvector.
      mask Display: disp('y = A*u')
  Mux : Mux  Inputs=2
  Mux1 : Mux
  Terminator : Terminator
  Terminator1 : Terminator
  Terminator2 : Terminator
  Cprop : Outport  InitialOutput=0
  wires:
  Fcn2/1 -> Mux1/4
  Fcn1/1 -> Mux1/3
  Fcn/1 -> Mux1/2
  Demux1/1 -> Mux1/1, Mux/1
  Mux/1 -> Fcn2/1, Fcn/1, Fcn1/1
  Demux/2 -> Mux/2
  ypow/1 -> Demux1/1
  x/1 -> Demux/1
  Mux1/1 -> Matrix Gain/1
  Matrix Gain/1 -> Cprop/1
  Demux1/2 -> Terminator/1
  Demux/3 -> Terminator1/1
  Demux/1 -> Terminator2/1

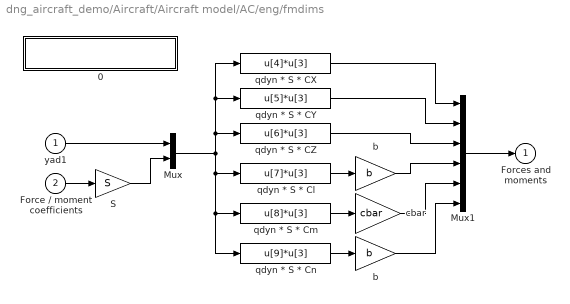
== system dng_aircraft_demo/Aircraft/Aircraft model/AC/eng/fmdims ==
  yad1 : Inport
  Force / moment coefficients : Inport  Port=2
  0 : Subsystem
      settings: OpenFcn=web('http://callisto.worldonline.nl/~rauw');
      mask Display: disp('FMDIMS\nM.O. Rauw, October 1997')
  Mux : Mux  Inputs=[3 6]
  Mux1 : Mux  Inputs=6
  S : Gain  Gain=S  SaturateOnIntegerOverflow=on
  b : Gain  Gain=b  SaturateOnIntegerOverflow=on
  "b " : Gain  Gain=b  SaturateOnIntegerOverflow=on
  cbar : Gain  Gain=cbar  SaturateOnIntegerOverflow=on
  qdyn * S * CX : Fcn  Expr=u[4]*u[3]
  qdyn * S * CY : Fcn  Expr=u[5]*u[3]
  qdyn * S * CZ : Fcn  Expr=u[6]*u[3]
  qdyn * S * Cl : Fcn  Expr=u[7]*u[3]
  qdyn * S * Cm : Fcn  Expr=u[8]*u[3]
  qdyn * S * Cn : Fcn  Expr=u[9]*u[3]
  Forces and moments : Outport  InitialOutput=0
  wires:
  b/1 -> Mux1/4
  qdyn * S * CZ/1 -> Mux1/3
  S/1 -> Mux/2
  qdyn * S * CY/1 -> Mux1/2
  qdyn * S * CX/1 -> Mux1/1
  yad1/1 -> Mux/1
  qdyn * S * Cn/1 -> "b "/1
  qdyn * S * Cm/1 -> cbar/1
  qdyn * S * Cl/1 -> b/1
  Mux/1 -> qdyn * S * Cn/1, qdyn * S * Cm/1, qdyn * S * Cl/1, qdyn * S * CY/1, qdyn * S * CX/1, qdyn * S * CZ/1
  Force / moment coefficients/1 -> S/1
  cbar/1 -> Mux1/5
  "b "/1 -> Mux1/6
  Mux1/1 -> Forces and moments/1

== system dng_aircraft_demo/Aircraft/Aircraft model/AC/eng/pow ==
  x : Inport
  uprop : Inport  Port=2
  yatm : Inport  Port=3
  0 : Subsystem
      settings: OpenFcn=web('http://callisto.worldonline.nl/~rauw');
      mask Display: disp('POWER\nM.O. Rauw, October 1997')
  Mux : Mux  Inputs=[12 2 5]
  Mux1 : Mux  Inputs=[19 1]
  Mux2 : Mux  Inputs=2
  P : Fcn  Expr=0.7355*(-326.5+0.00412*(u[14]+7.4)*(u[13]+2010)+(408.0-0.0965*u[13])*(1.0-u[15]/1.225))
  dpt : Fcn  Expr=0.08696 + 191.18*(u[20]/(0.5*u[15]*u[1]^3))
  ypow : Outport  InitialOutput=0
  wires:
  Mux1/1 -> dpt/1
  P/1 -> Mux1/2, Mux2/2
  Mux/1 -> Mux1/1, P/1
  x/1 -> Mux/1
  uprop/1 -> Mux/2
  yatm/1 -> Mux/3
  dpt/1 -> Mux2/1
  Mux2/1 -> ypow/1

== system dng_aircraft_demo/Aircraft/Aircraft model/AC/eqm/0 ==

== system dng_aircraft_demo/Aircraft/Aircraft model/AC/eqm/? ==

== system dng_aircraft_demo/Aircraft/Aircraft model/AC/eqm/ODE ==
  x : Inport
  Ftot : Inport  Port=2
  Mtot : Inport  Port=3
  yhlp : Inport  Port=4
  ybvel* : Inport  Port=5
  0 : Subsystem
      settings: OpenFcn=web('http://callisto.worldonline.nl/~rauw');
      mask Display: disp('12 Ordinary Differential\nEquations (level 4)\nM.O. Rauw')
  Eulerdot : Subsystem
      mask Type: Eulerdot
      mask Description:
      | Calculation of d(psi)/dt, d(theta)/dt,
      | and d(phi/dt)
      mask Help: web('http://callisto.worldonline.nl/~rauw');
      mask Display: disp('psi dot\ntheta dot\nphi dot')
  Mux : Mux  Inputs=[12 3 3 11]
  Mux1 : Mux  Inputs=[3 3 3 3]
  Vabdot : Subsystem  mask(Vabdot){m=GM1(10)}
      mask prompts: m "Mass of the aircraft [kg]:"
      mask help: Calculation of dV/dt, dalpha/dt, dbeta/dt.
      mask Help: web('http://callisto.worldonline.nl/~rauw');
      mask Display: disp('V dot\nalpha dot\nbeta dot')
  pqrdot : Subsystem
      mask Type: pqrdot
      mask Description: Calculation of dp/dt, dq/dt, and dr/dt
      mask Help: web('http://callisto.worldonline.nl/~rauw');
      mask Display: disp('p dot\nq dot\nr dot')
  xyHdot : Subsystem
      mask Type: xyHdot
      mask Description: Calculation of d(xe)/dt, d(ye)/dt, and dH/dt
      mask Help: web('http://callisto.worldonline.nl/~rauw');
      mask Display: disp('xe dot\nye dot\nH dot')
  xdot : Outport  InitialOutput=0
  wires:
  x/1 -> Mux/1
  Mtot/1 -> Mux/3
  Ftot/1 -> Mux/2
  Mux/1 -> pqrdot/1(upqr), Vabdot/1(uVab), Eulerdot/1(ueul), xyHdot/2(uxYH)
  ybvel*/1 -> xyHdot/1(ybvel*)
  yhlp/1 -> Mux/4
  xyHdot/1(yxyH) -> Mux1/4
  Eulerdot/1(yeul) -> Mux1/3
  pqrdot/1(ypqr) -> Mux1/2
  Vabdot/1(yVab) -> Mux1/1
  Mux1/1 -> xdot/1

== system dng_aircraft_demo/Aircraft/Aircraft model/AC/eqm/uvw ==
  yhlp : Inport
  x : Inport  Port=2
  0 : Subsystem
      settings: OpenFcn=web('http://callisto.worldonline.nl/~rauw');
      mask Display: disp('UVW\nM.O. Rauw, October 1997')
  Mux : Mux  Inputs=3
  Mux1 : Mux  Inputs=[12 11]
  u : Fcn  Expr=u[1]*u[13]*u[15]
  v : Fcn  Expr=u[1]*u[16]
  w : Fcn  Expr=u[1]*u[14]*u[15]
  ybvel : Outport  InitialOutput=0
  wires:
  Mux1/1 -> v/1, u/1, w/1
  yhlp/1 -> Mux1/2
  x/1 -> Mux1/1
  u/1 -> Mux/1
  v/1 -> Mux/2
  w/1 -> Mux/3
  Mux/1 -> ybvel/1

== system dng_aircraft_demo/Aircraft/Aircraft model/AC/eqm/xdotcorr ==
  xdot uncorrected : Inport
  yhlp : Inport  Port=2
  yatm : Inport  Port=3
  0 : Subsystem
      settings: OpenFcn=web('http://callisto.worldonline.nl/~rauw');
      mask Display: disp('XDOTCORR (Beaver)\nM.O. Rauw, October 1997')
  Demux : Demux  Outputs=12
  Mux1 : Mux  Inputs=12
  Mux2 : Mux  Inputs=[11 1 5]
  beta dot correction : Fcn  Expr=u[12] / (1 - (u[3]*u[13]*b*S*CYbdot)/(4*m))
  xdot corrected : Outport  InitialOutput=0
  wires:
  beta dot correction/1 -> Mux1/3
  yatm/1 -> Mux2/3
  Demux/1 -> Mux1/1
  Demux/2 -> Mux1/2
  Demux/4 -> Mux1/4
  Demux/5 -> Mux1/5
  Demux/6 -> Mux1/6
  Demux/7 -> Mux1/7
  Demux/8 -> Mux1/8
  Demux/9 -> Mux1/9
  Demux/10 -> Mux1/10
  Demux/11 -> Mux1/11
  Demux/12 -> Mux1/12
  Demux/3 -> Mux2/2
  xdot uncorrected/1 -> Demux/1
  Mux1/1 -> xdot corrected/1
  Mux2/1 -> beta dot correction/1
  yhlp/1 -> Mux2/1

== system dng_aircraft_demo/Aircraft/Aircraft model/AC/fms/0 ==

== system dng_aircraft_demo/Aircraft/Aircraft model/AC/fw/0 ==

== system dng_aircraft_demo/Aircraft/Aircraft model/AC/gr/0 ==

== system dng_aircraft_demo/Aircraft/Aircraft model/AC/hlp/0 ==

== system dng_aircraft_demo/Aircraft/Aircraft model/AC/out/0 ==

== system dng_aircraft_demo/Aircraft/Aircraft model/AC/out/accel ==
  Ftot : Inport
  Fgrav : Inport  Port=2
  0 : Subsystem
      settings: OpenFcn=web('http://callisto.worldonline.nl/~rauw');
      mask Display: disp('ACCEL\nM.O. Rauw, October 1997')
  Ax : Fcn  Expr=(u[1]-u[4])/(m*9.80665)
  Ay : Fcn  Expr=(u[2]-u[5])/(m*9.80665)
  Az : Fcn  Expr=(u[3]-u[6])/(m*9.80665)
  Mux : Mux  Inputs=6
  Mux1 : Mux  Inputs=[3 3]
  axk : Fcn  Expr=u[1]/(m*9.80665)
  ayk : Fcn  Expr=u[2]/(m*9.80665)
  azk : Fcn  Expr=u[3]/(m*9.80665)
  yacc : Outport  InitialOutput=0
  wires:
  ayk/1 -> Mux/5
  axk/1 -> Mux/4
  Mux1/1 -> ayk/1, azk/1, axk/1, Ay/1, Ax/1, Az/1
  Ax/1 -> Mux/1
  Ay/1 -> Mux/2
  Az/1 -> Mux/3
  azk/1 -> Mux/6
  Mux/1 -> yacc/1
  Fgrav/1 -> Mux1/2
  Ftot/1 -> Mux1/1

== system dng_aircraft_demo/Aircraft/Aircraft model/AC/out/fp ==
  x : Inport
  xdot : Inport  Port=2
  0 : Subsystem
      settings: OpenFcn=web('http://callisto.worldonline.nl/~rauw');
      mask Display: disp('FLPATH\nM.O. Rauw, October 1997')
  Mux : Mux  Inputs=[12 12]
  Mux1 : Mux
  Phi : Fcn  Expr=u[9]*cos(u[8]-alpha0)
  chi : Fcn  Expr=u[3]+u[7]
  fpa : Fcn  Expr=u[13]/9.80665
  gamma : Fcn  Expr=asin(u[24]/u[1])
  yfp : Outport  InitialOutput=0
  wires:
  xdot/1 -> Mux/2
  x/1 -> Mux/1
  Mux1/1 -> yfp/1
  Phi/1 -> Mux1/4
  chi/1 -> Mux1/3
  fpa/1 -> Mux1/2
  gamma/1 -> Mux1/1
  Mux/1 -> gamma/1, fpa/1, Phi/1, chi/1

== system dng_aircraft_demo/Aircraft/Aircraft model/AC/out/uvwdot ==
  note: V
  note: sin(beta)
  note: cos(beta)
  note: sin(alpha)
  note: cos(alpha)
  note: `
  x : Inport
  xdot : Inport  Port=2
  yhlp : Inport  Port=3
  0 : Subsystem
      settings: OpenFcn=web('http://callisto.worldonline.nl/~rauw');
      mask Display: disp('UVWDOT\nM.O. Rauw, October 1997')
  DeMux : Demux  Outputs=[1 1 1 1 7]
  Demux : Demux  Outputs=[1 11]
  Mux : Mux  Inputs=[1 1 1 1 1 12]
  Mux1 : Mux  Inputs=3
  Terminator : Terminator
  Terminator1 : Terminator
  u dot : Fcn  Expr=u[6]*u[1]*u[3] - u[5]*(u[7]*u[2]*u[3] + u[8]*u[1]*u[4])
  v dot : Fcn  Expr=u[6]*u[4] + u[5]*u[3]*u[8]
  wdot : Fcn  Expr=u[6]*u[2]*u[3] + u[5]*(u[7]*u[1]*u[3] - u[8]*u[2]*u[4])
  yuvw =  [udot; vdot; wdot] : Outport  InitialOutput=0
  wires:
  Demux/1 -> Mux/5
  DeMux/4 -> Mux/4
  DeMux/3 -> Mux/3
  yhlp/1 -> DeMux/1
  Mux1/1 -> yuvw =  [udot; vdot; wdot]/1
  x/1 -> Demux/1
  DeMux/2 -> Mux/2
  DeMux/1 -> Mux/1
  Mux/1 -> u dot/1, wdot/1, v dot/1
  xdot/1 -> Mux/6
  u dot/1 -> Mux1/1
  v dot/1 -> Mux1/2
  wdot/1 -> Mux1/3
  DeMux/5 -> Terminator/1
  Demux/2 -> Terminator1/1

== system dng_aircraft_demo/Aircraft/Aircraft model/AC/ad/ad1/0 ==

== system dng_aircraft_demo/Aircraft/Aircraft model/AC/ad/ad2/0 ==

== system dng_aircraft_demo/Aircraft/Aircraft model/AC/ad/ad3/0 ==

== system dng_aircraft_demo/Aircraft/Aircraft model/AC/ad/atm/0 ==

== system dng_aircraft_demo/Aircraft/Aircraft model/AC/ae/aero/0 ==

== system dng_aircraft_demo/Aircraft/Aircraft model/AC/ae/dl/0 ==

== system dng_aircraft_demo/Aircraft/Aircraft model/AC/ae/fmdims/0 ==

== system dng_aircraft_demo/Aircraft/Aircraft model/AC/eng/eng/0 ==

== system dng_aircraft_demo/Aircraft/Aircraft model/AC/eng/fmdims/0 ==

== system dng_aircraft_demo/Aircraft/Aircraft model/AC/eng/pow/0 ==

== system dng_aircraft_demo/Aircraft/Aircraft model/AC/eqm/ODE/0 ==

== system dng_aircraft_demo/Aircraft/Aircraft model/AC/eqm/ODE/Eulerdot ==
  note: ueul=[x;Ftot;Mtot;yhlp]
  note: yeul=[psi dot; theta dot; phi dot]
  ueul : Inport
  0 : Subsystem
      settings: OpenFcn=web('http://callisto.worldonline.nl/~rauw');
      mask Display: disp('EULERDOT\nM.O. Rauw, October 1997')
  Mux1 : Mux  Inputs=[29 1]
  Mux2 : Mux  Inputs=3
  phi dot : Fcn  Expr=u[4] + u[30]*u[26]
  psi dot : Fcn  Expr=(u[5]*u[28] + u[6]*u[29])/u[27]
  theta dot : Fcn  Expr=u[5]*u[29] - u[6]*u[28]
  yeul : Outport  InitialOutput=0
  wires:
  ueul/1 -> theta dot/1, Mux1/1, psi dot/1
  psi dot/1 -> Mux2/1, Mux1/2
  theta dot/1 -> Mux2/2
  Mux2/1 -> yeul/1
  phi dot/1 -> Mux2/3
  Mux1/1 -> phi dot/1

== system dng_aircraft_demo/Aircraft/Aircraft model/AC/eqm/ODE/Vabdot ==
  note: yVab=[V dot;alpha dot;beta dot]
  note: uVab=[x;Ftot;Mtot;yhlp]
  uVab : Inport
  0 : Subsystem
      settings: OpenFcn=web('http://callisto.worldonline.nl/~rauw');
      mask Display: disp('VABDOT\nM.O. Rauw, October 1997')
  Mux2 : Mux  Inputs=3
  V dot : Fcn  Expr=(u[13]*u[19]*u[21]+u[14]*u[22]+u[15]*u[20]*u[21])/m
  alpha dot : Fcn  Expr=(-u[13]*u[20]+u[15]*u[19])/(m*u[1]*u[21]) - u[23]*(u[4]*u[19]+u[6]*u[20]) + u[5]
  beta dot : Fcn  Expr=(-u[13]*u[19]*u[22]+u[14]*u[21]-u[15]*u[20]*u[22])/(m*u[1]) + u[4]*u[20] - u[6]*u[19]
  yVab : Outport  InitialOutput=0
  wires:
  beta dot/1 -> Mux2/3
  V dot/1 -> Mux2/1
  alpha dot/1 -> Mux2/2
  uVab/1 -> alpha dot/1, beta dot/1, V dot/1
  Mux2/1 -> yVab/1

== system dng_aircraft_demo/Aircraft/Aircraft model/AC/eqm/ODE/pqrdot ==
  note: ytmp = [L; M; N; p^2; pq; pr; q^2; qr; r^2]
  note: upqr=[x;Ftot;Mtot;yhlp]
  note: ypqr=[p dot;q dot;r dot]
  note: ytmp
  note: Here: ypqr = GM2*ytmp
  note: [L M N]'
  note: [p q r]'
  upqr : Inport
  0 : Subsystem
      settings: OpenFcn=web('http://callisto.worldonline.nl/~rauw');
      mask Display: disp('PQRDOT\nM.O. Rauw, October 1997')
  Demux : Demux  Outputs=[3 3 9 3 11]
  Fcn : Fcn  Expr=u[1]^2
  Fcn1 : Fcn  Expr=u[1]*u[2]
  Fcn2 : Fcn  Expr=u[1]*u[3]
  Fcn3 : Fcn  Expr=u[2]^2
  Fcn4 : Fcn  Expr=u[2]*u[3]
  Fcn5 : Fcn  Expr=u[3]^2
  Matrix Gain : StateSpace  A=A  B=B  C=C  D=D  mask(Matrix Gain){@1=GM2}
      mask prompts: @1 "Gain matrix:"
      mask help: Matrix Gain
      mask init:
      | A = []; B = []; C = []; D = @1;
      mask Help: This block implements an matrix gain.\nThe matrix dimensions must be in accordance\nwith the dimension of the inputvector.
      mask Display: disp('y = A*u')
  Mux : Mux  Inputs=[3 1 1 1 1 1 1]
  Terminator1 : Terminator
  Terminator2 : Terminator
  Terminator3 : Terminator
  ypqr : Outport  InitialOutput=0
  wires:
  Mux/1 -> Matrix Gain/1
  Matrix Gain/1 -> ypqr/1
  Fcn5/1 -> Mux/7
  Fcn4/1 -> Mux/6
  Fcn3/1 -> Mux/5
  Fcn2/1 -> Mux/4
  Fcn1/1 -> Mux/3
  Fcn/1 -> Mux/2
  Demux/4 -> Mux/1
  Demux/2 -> Fcn3/1, Fcn5/1, Fcn4/1, Fcn2/1, Fcn/1, Fcn1/1
  Demux/3 -> Terminator1/1
  Demux/5 -> Terminator2/1
  Demux/1 -> Terminator3/1
  upqr/1 -> Demux/1

== system dng_aircraft_demo/Aircraft/Aircraft model/AC/eqm/ODE/xyHdot ==
  note: uxyH=[x;Ftot;Mtot;yhlp]
  note: yxyH=[xe dot; ye dot; H dot]
  ybvel* : Inport
  uxYH : Inport  Port=2
  0 : Subsystem
      settings: OpenFcn=web('http://callisto.worldonline.nl/~rauw');
      mask Display: disp('XYHDOT\nM.O. Rauw, October 1997')
  H dot : Fcn  Expr=u[30]*u[26] - (u[31]*u[28]+u[32]*u[29])*u[27]
  Mux2 : Mux  Inputs=[29 3]
  Mux3 : Mux  Inputs=2
  Mux4 : Mux  Inputs=[29 2]
  Mux5 : Mux  Inputs=3
  tmp1 : Fcn  Expr=u[30]*u[27] + (u[31]*u[28]+u[32]*u[29])*u[26]
  tmp2 : Fcn  Expr=u[31]*u[29] - u[32]*u[28]
  xe dot : Fcn  Expr=u[30]*u[25] - u[31]*u[24]
  ye dot : Fcn  Expr=u[30]*u[24] + u[31]*u[25]
  yxyH : Outport  InitialOutput=0
  wires:
  uxYH/1 -> Mux2/1, Mux4/1
  ybvel*/1 -> Mux2/2
  Mux3/1 -> Mux4/2
  Mux2/1 -> tmp1/1, tmp2/1, H dot/1
  Mux4/1 -> xe dot/1, ye dot/1
  Mux5/1 -> yxyH/1
  ye dot/1 -> Mux5/2
  tmp2/1 -> Mux3/2
  xe dot/1 -> Mux5/1
  H dot/1 -> Mux5/3
  tmp1/1 -> Mux3/1

== system dng_aircraft_demo/Aircraft/Aircraft model/AC/eqm/uvw/0 ==

== system dng_aircraft_demo/Aircraft/Aircraft model/AC/eqm/xdotcorr/0 ==

== system dng_aircraft_demo/Aircraft/Aircraft model/AC/out/accel/0 ==

== system dng_aircraft_demo/Aircraft/Aircraft model/AC/out/fp/0 ==

== system dng_aircraft_demo/Aircraft/Aircraft model/AC/out/uvwdot/0 ==

== system dng_aircraft_demo/Aircraft/Aircraft model/AC/eqm/ODE/Eulerdot/0 ==

== system dng_aircraft_demo/Aircraft/Aircraft model/AC/eqm/ODE/Vabdot/0 ==

== system dng_aircraft_demo/Aircraft/Aircraft model/AC/eqm/ODE/pqrdot/0 ==

== system dng_aircraft_demo/Aircraft/Aircraft model/AC/eqm/ODE/xyHdot/0 ==
